simulink model "discrete"  (R2015a)
settings: Solver=ode3  StartTime=0.0  StopTime=5  FixedStep=0.001  RelTol=1e-3
values from neighbouring files (symbols this model uses):
  anpha_0 = 5    [ANN_params.m]    (also in furuta.m)
  beta0 = 5.8*10^(-4)    (= 0.00058)    [ANN_params.m]    (also in furuta.m)
  beta1 = 1.4142*10^(-3)    (= 0.0014142)    [ANN_params.m]    (also in furuta.m)
  c = 10    [ANN_params.m]
  g = 9.81    [ANN_params.m]    (also in furuta.m)
  J0 = 4.4*10^(-3)    (= 0.0044)    [ANN_params.m]    (also in furuta.m)
  J1 = 5.5026*10^(-4)    (= 0.00055026)    [ANN_params.m]    (also in furuta.m)
  k = 3    [ANN_params.m]
  L0 = 0.157    [ANN_params.m]    (also in furuta.m)
  L1 = 0.133    [ANN_params.m]    (also in furuta.m)
  m1 = 0.078    [ANN_params.m]    (also in furuta.m = 0.0933)
  muy = 0.99    [ANN_params.m]    (also in furuta.m)
  theta_0 = 0    [ANN_params.m]    (also in furuta.m)
settings Model: Creator=chech  LastModifiedBy=chech
settings SolverCC: ZeroCrossAlgorithm=Adaptive  AlgebraicLoopSolver=LineSearch

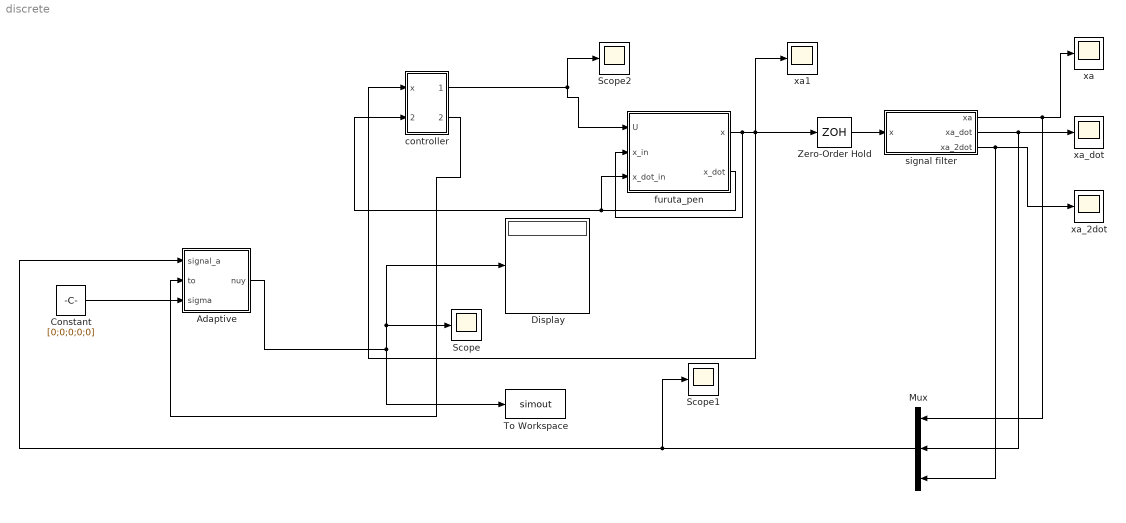
== system discrete ==
  Adaptive : Subsystem
  Constant : Constant  Value=[0;0;0;0;0]
  Display : Display
  Mux : Mux  Inputs=3
  Scope : Scope
      settings: TimeRange=5  YMin=-600000  YMax=200000  SaveName=ScopeData3
  Scope1 : Scope
      settings: YMin=-6  YMax=2  SaveName=ScopeData9
  Scope2 : Scope
      settings: SaveName=ScopeData12
  To Workspace : ToWorkspace  VariableName=simout  SaveFormat=Timeseries  SampleTime=-1
  Zero-Order Hold : ZeroOrderHold  SampleTime=0.001
  controller : Subsystem
  furuta_pen : Subsystem
  signal filter : Subsystem
  xa : Scope
      settings: TimeRange=5  YMin=0  YMax=32.5
  xa1 : Scope
      settings: TimeRange=5  YMin=0  YMax=55  SaveName=ScopeData20
  xa_2dot : Scope
      settings: TimeRange=5  YMin=-0.15  YMax=0.25  SaveName=ScopeData2
  xa_dot : Scope
      settings: TimeRange=5  YMin=-1.9  YMax=0.1
  wires:
  signal filter/1(xa) -> Mux/1, xa/1
  signal filter/2(xa_dot) -> Mux/2, xa_dot/1
  Zero-Order Hold/1 -> signal filter/1(x)
  signal filter/3(xa_2dot) -> Mux/3, xa_2dot/1
  Mux/1 -> Scope1/1, Adaptive/1(signal_a)
  furuta_pen/2(x_dot) -> controller/2(x_dot), furuta_pen/3(x_dot_in)
  furuta_pen/1(x) -> controller/1(x), xa1/1, Zero-Order Hold/1, furuta_pen/2(x_in)
  Adaptive/1(nuy) -> Display/1, Scope/1, To Workspace/1
  controller/1(Out1) -> furuta_pen/1(U), Scope2/1
  controller/2(Out2) -> Adaptive/2(to)
  Constant/1 -> Adaptive/3(sigma)

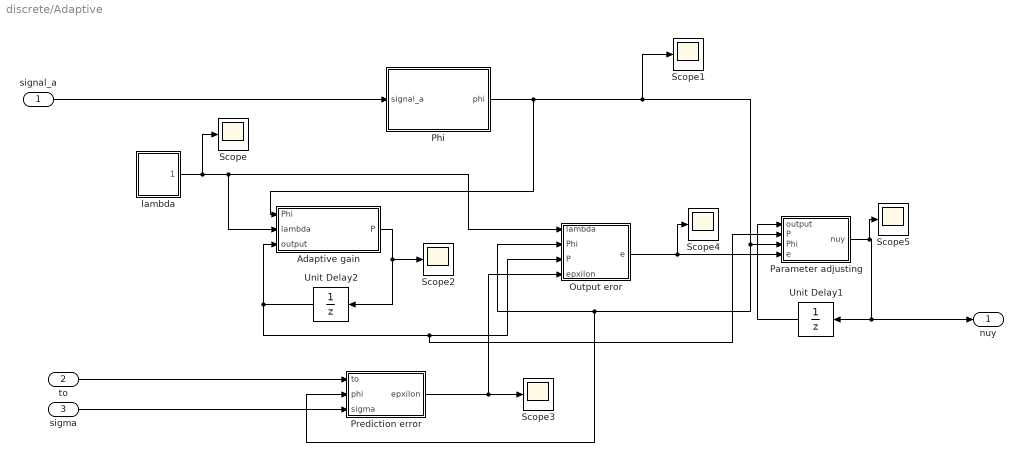
== system discrete/Adaptive ==
  signal_a : Inport
  to : Inport  Port=2
  sigma : Inport  Port=3
  Adaptive gain : Subsystem
  Output eror : Subsystem
  Parameter adjusting : Subsystem
  Phi : Subsystem
  Prediction error : Subsystem
  Scope{,1..5} (6 alike) : Scope
      Scope settings: YMin=1  YMax=1  SaveName=ScopeData10
      Scope1 settings: TimeRange=5  SaveName=ScopeData11
      Scope2 settings: YMin=8.6e-06  YMax=9.6e-06  SaveName=ScopeData13
      Scope3 settings: SaveName=ScopeData14
      Scope4 settings: SaveName=ScopeData15
      Scope5 settings: SaveName=ScopeData16
  Unit Delay1 : UnitDelay  InitialCondition=[1;1;1;1;1]  SampleTime=0.001
  Unit Delay2 : UnitDelay  InitialCondition=eye(5)  SampleTime=0.001
  lambda : Subsystem
  nuy : Outport
  wires:
  Unit Delay1/1 -> Parameter adjusting/1(output)
  Output eror/1(e) -> Scope4/1, Parameter adjusting/4(e)
  Adaptive gain/1(P) -> Scope2/1, Unit Delay2/1
  Unit Delay2/1 -> Parameter adjusting/2(P), Output eror/3(P), Adaptive gain/3(output)
  lambda/1(lambda) -> Scope/1, Adaptive gain/2(lambda), Output eror/1(lambda)
  Prediction error/1(epxilon) -> Scope3/1, Output eror/4(epxilon)
  signal_a/1 -> Phi/1(signal_a)
  Phi/1(phi) -> Adaptive gain/1(Phi), Scope1/1, Prediction error/2(phi), Output eror/2(Phi), Parameter adjusting/3(Phi)
  to/1 -> Prediction error/1(to)
  sigma/1 -> Prediction error/3(sigma)
  Parameter adjusting/1(nuy) -> Scope5/1, nuy/1, Unit Delay1/1

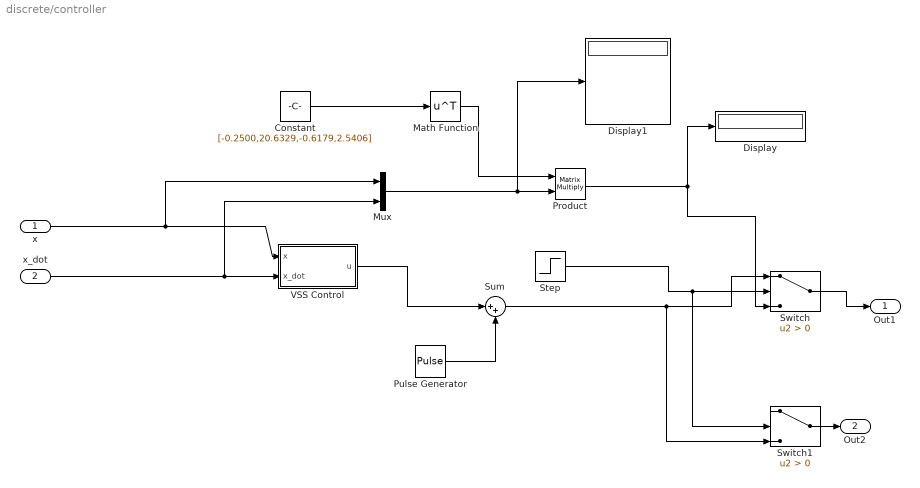
== system discrete/controller ==
  x : Inport
  x_dot : Inport  Port=2
  Constant : Constant  Value=[-0.2500,20.6329,-0.6179,2.5406]
  Display : Display
  Display1 : Display
  Math Function : Math  Operator=transpose  SaturateOnIntegerOverflow=on
  Mux : Mux  Inputs=2
  Product : Product  Multiplication=Matrix(*)
  Pulse Generator : DiscretePulseGenerator  PulseType=Time based  Period=1  PulseWidth=5
  Step : Step  Time=6  SampleTime=0
  Sum : Sum  Inputs=|++
  Switch : Switch  Criteria=u2 > Threshold
  Switch1 : Switch  Criteria=u2 > Threshold
  VSS Control : Subsystem
  Out1 : Outport
  Out2 : Outport  Port=2
  wires:
  Sum/1 -> Switch/1, Switch1/3
  Pulse Generator/1 -> Sum/2
  x_dot/1 -> Mux/2, VSS Control/2(x_dot)
  x/1 -> Mux/1, VSS Control/1(x)
  VSS Control/1(u) -> Sum/1
  Step/1 -> Switch1/2, Switch/2
  Switch/1 -> Out1/1
  Product/1 -> Switch/3, Display/1
  Mux/1 -> Display1/1, Product/2
  Constant/1 -> Math Function/1
  Math Function/1 -> Product/1
  Switch1/1 -> Out2/1

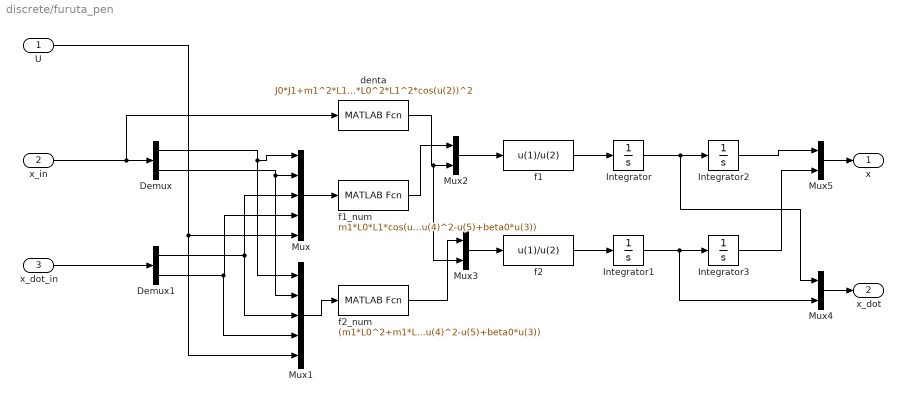
== system discrete/furuta_pen ==
  U : Inport
  x_in : Inport  Port=2
  x_dot_in : Inport  Port=3
  Demux : Demux  Outputs=2
  Demux1 : Demux  Outputs=2
  Integrator : Integrator
  Integrator1 : Integrator
  Integrator2 : Integrator  InitialCondition=theta_0*pi/180
  Integrator3 : Integrator  InitialCondition=anpha_0/180*pi
  Mux : Mux  Inputs=5
  Mux1 : Mux  Inputs=5
  Mux{2..5} (4 alike) : Mux  Inputs=2
  denta : MATLABFcn  MATLABFcn=J0*J1+m1^2*L1^4*sin(u(2))^2+m1^2*L0^2*L1^2+J0*m1*L1^2+J1*m1*L0^2+J1*m1*L1^2*sin(u(2))^2-m1^2*L0^2*L1^2*cos(u(2))^2  OutputDimensions=1
  f1 : MATLABFcn  MATLABFcn=u(1)/u(2)  OutputDimensions=1
  f1_num : MATLABFcn  MATLABFcn=m1*L0*L1*cos(u(2))*(0.5*m1*L1^2*sin(2*u(2))*u(3)^2+m1*g*L1*sin(u(2))-beta1*u(4))-(m1*L1^2+J1)*(m1*L1^2*sin(2*u(2))*u(3)*u(4)+m1*L0*L1*sin(u(2))*u(4)^2-u(5)+beta0*u(3))  OutputDimensions=1
  f2 : MATLABFcn  MATLABFcn=u(1)/u(2)  OutputDimensions=1
  f2_num : MATLABFcn  MATLABFcn=(m1*L0^2+m1*L1^2*sin(u(2))^2+J0)*(0.5*m1*L1^2*sin(2*u(2))*u(3)^2+m1*g*L1*sin(u(2))-beta1*u(4))-m1*L0*L1*cos(u(2))*(m1*L1^2*sin(2*u(2))*u(3)*u(4)+m1*L0*L1*sin(u(2))*u(4)^2-u(5)+beta0*u(3))  OutputDimensions=1
  x : Outport
  x_dot : Outport  Port=2
  wires:
  x_in/1 -> Demux/1, denta/1
  Mux/1 -> f1_num/1
  Mux1/1 -> f2_num/1
  denta/1 -> Mux3/2, Mux2/2
  f1_num/1 -> Mux2/1
  f2_num/1 -> Mux3/1
  f1/1 -> Integrator/1
  f2/1 -> Integrator1/1
  Integrator/1 -> Mux4/1, Integrator2/1
  Integrator1/1 -> Mux4/2, Integrator3/1
  Mux4/1 -> x_dot/1
  Mux5/1 -> x/1
  Integrator2/1 -> Mux5/1
  Integrator3/1 -> Mux5/2
  U/1 -> Mux1/5, Mux/5
  x_dot_in/1 -> Demux1/1
  Demux/1 -> Mux1/1, Mux/1
  Demux/2 -> Mux1/2, Mux/2
  Demux1/2 -> Mux1/4, Mux/4
  Demux1/1 -> Mux1/3, Mux/3
  Mux2/1 -> f1/1
  Mux3/1 -> f2/1

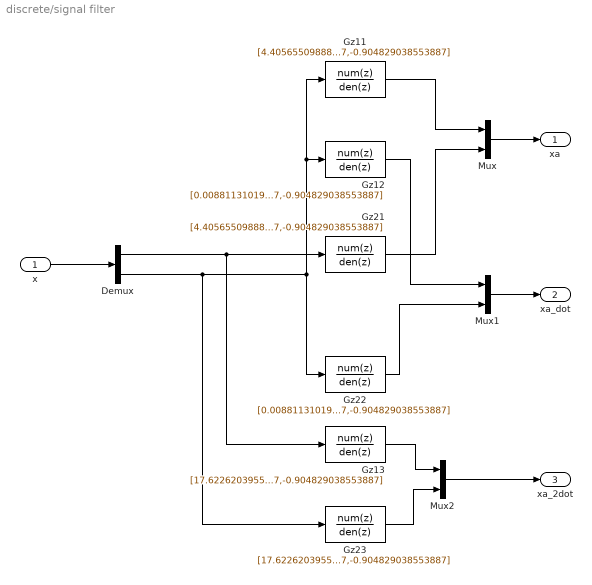
== system discrete/signal filter ==
  x : Inport
  Demux : Demux  Outputs=2
  Gz11 : DiscreteTransferFcn  Numerator=[4.40565509888493e-06,1.32169652966548e-05,1.32169652966548e-05,4.40565509888493e-06]  Denominator=[1,-2.90163934426229,2.80650362805697,-0.904829038553887]  SampleTime=0.001
  Gz12 : DiscreteTransferFcn  Numerator=[0.00881131019776986,0.00881131019776986,-0.00881131019776986,-0.00881131019776986]  Denominator=[1,-2.90163934426229,2.80650362805697,-0.904829038553887]  SampleTime=0.001
  Gz13 : DiscreteTransferFcn  Numerator=[17.6226203955397,-17.6226203955397,-17.6226203955397,17.6226203955397]  Denominator=[1,-2.90163934426229,2.80650362805697,-0.904829038553887]  SampleTime=0.001
  Gz21 : DiscreteTransferFcn  Numerator=[4.40565509888493e-06,1.32169652966548e-05,1.32169652966548e-05,4.40565509888493e-06]  Denominator=[1,-2.90163934426229,2.80650362805697,-0.904829038553887]  SampleTime=0.001
  Gz22 : DiscreteTransferFcn  Numerator=[0.00881131019776986,0.00881131019776986,-0.00881131019776986,-0.00881131019776986]  Denominator=[1,-2.90163934426229,2.80650362805697,-0.904829038553887]  SampleTime=0.001
  Gz23 : DiscreteTransferFcn  Numerator=[17.6226203955397,-17.6226203955397,-17.6226203955397,17.6226203955397]  Denominator=[1,-2.90163934426229,2.80650362805697,-0.904829038553887]  SampleTime=0.001
  Mux : Mux  Inputs=2
  Mux1 : Mux  Inputs=2
  Mux2 : Mux  Inputs=2
  xa : Outport
  xa_dot : Outport  Port=2
  xa_2dot : Outport  Port=3
  wires:
  x/1 -> Demux/1
  Gz12/1 -> Mux1/1
  Demux/2 -> Gz23/1, Gz22/1, Gz21/1
  Mux1/1 -> xa_dot/1
  Gz22/1 -> Mux1/2
  Gz11/1 -> Mux/1
  Gz21/1 -> Mux/2
  Mux/1 -> xa/1
  Demux/1 -> Gz13/1, Gz11/1, Gz12/1
  Gz13/1 -> Mux2/1
  Mux2/1 -> xa_2dot/1
  Gz23/1 -> Mux2/2

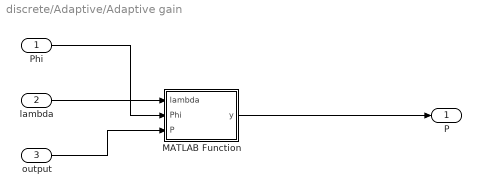
== system discrete/Adaptive/Adaptive gain ==
  Phi : Inport
  lambda : Inport  Port=2
  output : Inport  Port=3
  MATLAB Function : MATLAB Function  TreatAsAtomicUnit=on
  P : Outport
  wires:
  output/1 -> MATLAB Function/3(P)
  lambda/1 -> MATLAB Function/1(lambda)
  Phi/1 -> MATLAB Function/2(Phi)
  MATLAB Function/1(y) -> P/1

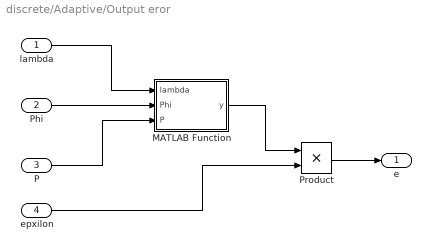
== system discrete/Adaptive/Output eror ==
  lambda : Inport
  Phi : Inport  Port=2
  P : Inport  Port=3
  epxilon : Inport  Port=4
  MATLAB Function : MATLAB Function  TreatAsAtomicUnit=on
  Product : Product
  e : Outport
  wires:
  lambda/1 -> MATLAB Function/1(lambda)
  Phi/1 -> MATLAB Function/2(Phi)
  P/1 -> MATLAB Function/3(P)
  MATLAB Function/1(y) -> Product/1
  epxilon/1 -> Product/2
  Product/1 -> e/1

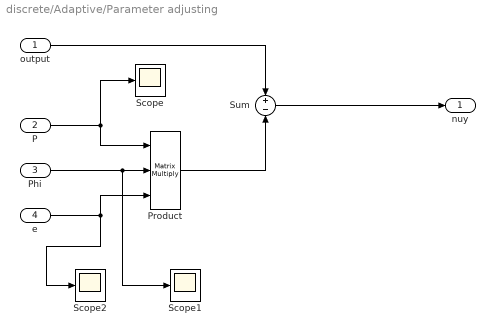
== system discrete/Adaptive/Parameter adjusting ==
  output : Inport
  P : Inport  Port=2
  Phi : Inport  Port=3
  e : Inport  Port=4
  Product : Product  Inputs=3  Multiplication=Matrix(*)
  Scope : Scope
      settings: SaveName=ScopeData17
  Scope1 : Scope
      settings: YMin=-3.5  YMax=2.5  SaveName=ScopeData18
  Scope2 : Scope
      settings: YMin=-4  YMax=7  SaveName=ScopeData19
  Sum : Sum  Inputs=+-
  nuy : Outport
  wires:
  P/1 -> Scope/1, Product/1
  Phi/1 -> Scope1/1, Product/2
  Product/1 -> Sum/2
  output/1 -> Sum/1
  Sum/1 -> nuy/1
  e/1 -> Product/3, Scope2/1

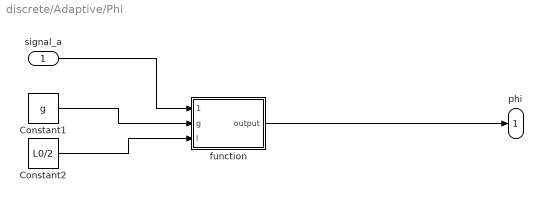
== system discrete/Adaptive/Phi ==
  signal_a : Inport
  Constant1 : Constant  Value=g
  Constant2 : Constant  Value=L0/2
  function : MATLAB Function  TreatAsAtomicUnit=on
  phi : Outport
  wires:
  function/1(output) -> phi/1
  signal_a/1 -> function/1(signal_a)
  Constant2/1 -> function/3(l)
  Constant1/1 -> function/2(g)

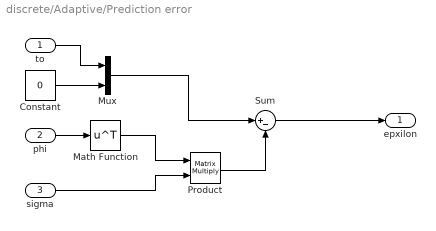
== system discrete/Adaptive/Prediction error ==
  to : Inport
  phi : Inport  Port=2
  sigma : Inport  Port=3
  Constant : Constant  Value=0
  Math Function : Math  Operator=transpose  SaturateOnIntegerOverflow=on
  Mux : Mux  Inputs=2
  Product : Product  Multiplication=Matrix(*)
  Sum : Sum  Inputs=|+-
  epxilon : Outport
  wires:
  Constant/1 -> Mux/2
  to/1 -> Mux/1
  phi/1 -> Math Function/1
  Math Function/1 -> Product/1
  sigma/1 -> Product/2
  Mux/1 -> Sum/1
  Product/1 -> Sum/2
  Sum/1 -> epxilon/1

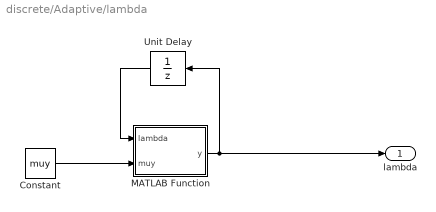
== system discrete/Adaptive/lambda ==
  Constant : Constant  Value=muy
  MATLAB Function : MATLAB Function  TreatAsAtomicUnit=on
  Unit Delay : UnitDelay  SampleTime=-1
  lambda : Outport
  wires:
  Constant/1 -> MATLAB Function/2(muy)
  MATLAB Function/1(y) -> lambda/1, Unit Delay/1
  Unit Delay/1 -> MATLAB Function/1(lambda)

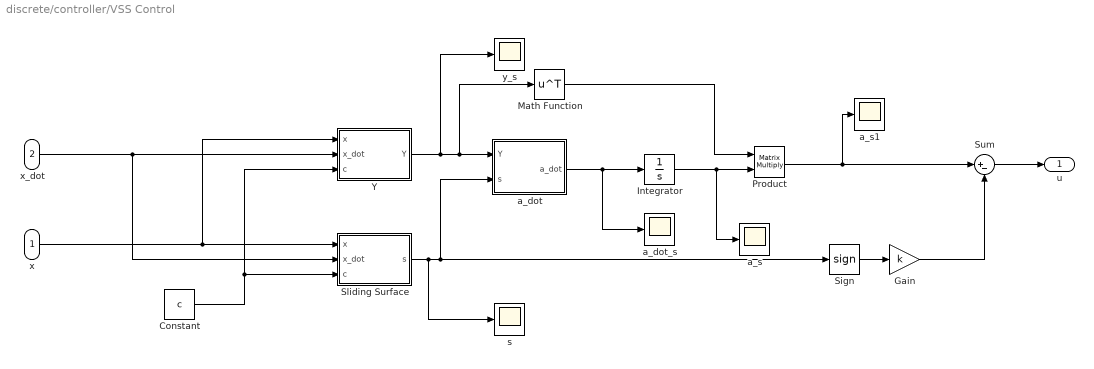
== system discrete/controller/VSS Control ==
  x : Inport
  x_dot : Inport  Port=2
  Constant : Constant  Value=c
  Gain : Gain  Gain=k
  Integrator : Integrator  InitialCondition=[0.5;0.5;0.5;0.5]
  Math Function : Math  Operator=transpose  SaturateOnIntegerOverflow=on
  Product : Product  Multiplication=Matrix(*)
  Sign : Signum
  Sliding Surface : MATLAB Function  TreatAsAtomicUnit=on
  Sum : Sum  Inputs=|+-
  Y : MATLAB Function  TreatAsAtomicUnit=on
  a_dot : MATLAB Function  TreatAsAtomicUnit=on
  a_dot_s : Scope
      settings: YMin=-0.175  YMax=0.175  SaveName=ScopeData6
  a_s : Scope
      settings: YMin=0.491  YMax=0.504  SaveName=ScopeData7
  a_s1 : Scope
      settings: YMin=0.491  YMax=0.504  SaveName=ScopeData8
  s : Scope
      settings: YMin=-0.175  YMax=0.175  SaveName=ScopeData5
  y_s : Scope
      settings: YMin=-0.175  YMax=0.175  SaveName=ScopeData4
  u : Outport
  wires:
  x_dot/1 -> Sliding Surface/2(x_dot), Y/2(x_dot)
  x/1 -> Y/1(x), Sliding Surface/1(x)
  Constant/1 -> Sliding Surface/3(c), Y/3(c)
  a_dot/1(a_dot) -> a_dot_s/1, Integrator/1
  Y/1(Y) -> y_s/1, Math Function/1, a_dot/1(Y)
  Sliding Surface/1(s) -> s/1, a_dot/2(s), Sign/1
  Math Function/1 -> Product/1
  Integrator/1 -> a_s/1, Product/2
  Product/1 -> a_s1/1, Sum/1
  Sign/1 -> Gain/1
  Gain/1 -> Sum/2
  Sum/1 -> u/1

== matlab function discrete/Adaptive/Output eror/MATLAB Function ==
  data: lambda input; y output; Phi input size=[5 2]; P input size=[5 5]
function y = fcn(lambda, Phi, P)
%#codegen
den = lambda + trace(Phi'*P*Phi);
y = 1/den;

== matlab function discrete/Adaptive/Phi/function ==
  data: signal_a input size=6; output output; g input; l input
function output = fcn(signal_a,g,l)
%#codegen
theta = signal_a(1:2);
thetaDot = signal_a(3:4);
theta2Dot = signal_a(5:6);

output = [theta2Dot(1),sin(theta(2))^2*theta2Dot(1)+sin(2*theta(2))*thetaDot(1)*thetaDot(2),l*(sin(theta(2))*thetaDot(2)^2-cos(theta(2))*theta2Dot(2)),thetaDot(1),0;
    0,theta2Dot(2)-sin(theta(2))*cos(theta(2))*thetaDot(1)^2,-l*cos(theta(2))*theta2Dot(1)-g*sin(theta(2)),0,thetaDot(2)]';

== matlab function discrete/Adaptive/Adaptive gain/MATLAB Function ==
  data: lambda input size=1; y output; Phi input size=[5 2]; P input size=[5 5]
function y = fcn(lambda, Phi, P)
%#codegen
num = P*Phi*Phi'*P;
den = lambda + trace(Phi'*P*Phi);
y = 1/lambda*(P-num/den);

== matlab function discrete/Adaptive/lambda/MATLAB Function ==
  data: lambda input; y output; muy input
function y = fcn(lambda,muy)
%#codegen

y = (1-muy)*lambda+muy;

== matlab function discrete/controller/VSS Control/Sliding Surface ==
  data: x input size=2; s output size=1; x_dot input size=2; c input size=1
function s = fcn(x,x_dot,c)
%#codegen
s = x_dot(2)+c*x(2);

== matlab function discrete/controller/VSS Control/Y ==
  data: x input size=2; Y output; x_dot input size=2; c input size=1
function Y = fnc(x,x_dot,c)
%#codegen

Y = [-c*x_dot(2);x_dot(2);x(2);x_dot(1)];

== matlab function discrete/controller/VSS Control/a_dot ==
  data: Y input size=4; s input size=1; a_dot output
function a_dot = fnc(Y,s)
%#codegen
ro = 100*eye(4);
a_dot = -ro^(-1)*Y*s;
